simulink model "dry +no way scenario 1"  (R2025a)
settings: Solver=VariableStepAuto  StartTime=0.0  StopTime=10.0  RelTol=1e-3
libraries: SignalEditorBlockLib x5
settings Model: Creator=josik  LastModifiedBy=josik

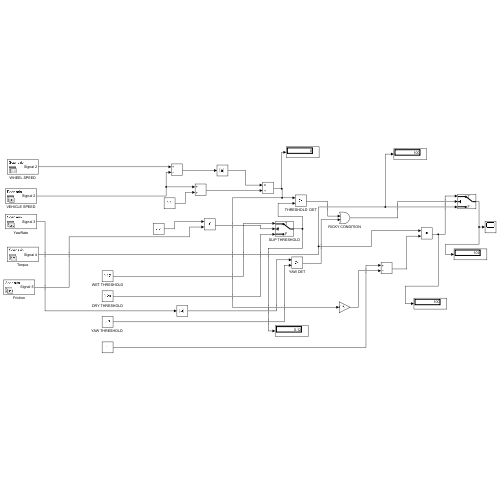
[thumbnail: Simulink's stored preview of the top-level diagram]
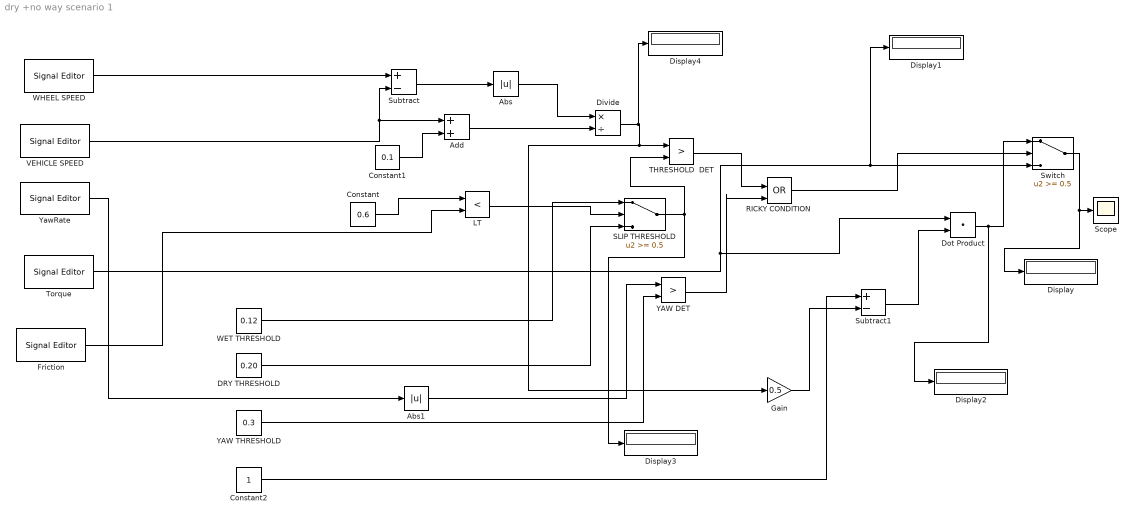
== system dry +no way scenario 1 ==
  Abs : Abs  SaturateOnIntegerOverflow=off
  Abs1 : Abs  SaturateOnIntegerOverflow=off
  Add : Sum
  Constant : Constant  Value=0.6
  Constant1 : Constant  Value=0.1
  Constant2 : Constant
  DRY THRESHOLD : Constant  Value=0.20
  Display{,1..4} (5 alike) : Display
  Divide : Product  Inputs=*/
  Dot Product : DotProduct  OutDataTypeStr=Inherit: Inherit via internal rule
  Friction : SignalEditorBlockLib/Signal Editor  FileName=signal 5 sc 3.mat  ActiveScenario=Scenario  ActiveSignal=Signal 5  IsBus=off  OutputBusObjectStr=Bus: BusObject  SampleTime=0  ZeroCross=off  OutputAfterFinalValue=Setting to zero  Unit=inherit  PreserveSignalName=on  ApplySigPropsToAllScenarios=on  ApplySigPropsToAllSignals=off  SignalPropertySource=Dialog parameters
  Gain : Gain  Gain=0.5
  LT : RelationalOperator  Operator=<  OutDataTypeStr=boolean  RndMeth=Simplest  InputSameDT=off
  RICKY CONDITION : Logic  Operator=OR  IconShape=distinctive  AllPortsSameDT=off  OutDataTypeStr=boolean
  SLIP THRESHOLD : Switch  Threshold=0.5  SaturateOnIntegerOverflow=off  InputSameDT=off
  Scope : Scope
      settings: ActiveDisplayYMinimum=0.26299668874172188  ActiveDisplayYMaximum=0.97077814569536425
  Subtract : Sum  Inputs=+-
  Subtract1 : Sum  Inputs=+-
  Switch : Switch  Threshold=0.5  SaturateOnIntegerOverflow=off  InputSameDT=off
  THRESHOLD  DET : RelationalOperator  Operator=>  OutDataTypeStr=boolean  RndMeth=Simplest  InputSameDT=off
  Torque : SignalEditorBlockLib/Signal Editor  FileName=signal 4 sc 3.mat  ActiveScenario=Scenario  ActiveSignal=Signal 4  IsBus=off  OutputBusObjectStr=Bus: BusObject  SampleTime=0  ZeroCross=off  OutputAfterFinalValue=Setting to zero  Unit=inherit  PreserveSignalName=on  ApplySigPropsToAllScenarios=on  ApplySigPropsToAllSignals=off  SignalPropertySource=Dialog parameters
  VEHICLE SPEED : SignalEditorBlockLib/Signal Editor  FileName=signal 2 sc 3.mat  ActiveScenario=Scenario  ActiveSignal=Signal 2  IsBus=off  OutputBusObjectStr=Bus: BusObject  SampleTime=0  ZeroCross=off  OutputAfterFinalValue=Setting to zero  Unit=inherit  PreserveSignalName=on  ApplySigPropsToAllScenarios=on  ApplySigPropsToAllSignals=off  SignalPropertySource=Dialog parameters
  WET THRESHOLD : Constant  Value=0.12
  WHEEL SPEED : SignalEditorBlockLib/Signal Editor  FileName=signal 2 sc 3.mat  ActiveScenario=Scenario  ActiveSignal=Signal 2  IsBus=off  OutputBusObjectStr=Bus: BusObject  SampleTime=0  ZeroCross=off  OutputAfterFinalValue=Setting to zero  Unit=inherit  PreserveSignalName=on  ApplySigPropsToAllScenarios=on  ApplySigPropsToAllSignals=off  SignalPropertySource=Dialog parameters
  YAW DET : RelationalOperator  Operator=>  OutDataTypeStr=boolean  RndMeth=Simplest  InputSameDT=off
  "YAW THRESHOLD " : Constant  Value=0.3
  YawRate : SignalEditorBlockLib/Signal Editor  FileName=signal 3 sc 3.mat  ActiveScenario=Scenario  ActiveSignal=Signal 3  IsBus=off  OutputBusObjectStr=Bus: BusObject  SampleTime=0  ZeroCross=off  OutputAfterFinalValue=Setting to zero  Unit=inherit  PreserveSignalName=on  ApplySigPropsToAllScenarios=on  ApplySigPropsToAllSignals=off  SignalPropertySource=Dialog parameters
  wires:
  Abs/1 -> Divide/1
  LT/1 -> SLIP THRESHOLD/2
  THRESHOLD  DET/1 -> RICKY CONDITION/1
  SLIP THRESHOLD/1 -> THRESHOLD  DET/2, Display3/1
  Constant/1 -> LT/1
  VEHICLE SPEED/1 -> Subtract/2, Add/1
  DRY THRESHOLD/1 -> SLIP THRESHOLD/3
  Gain/1 -> Subtract1/2
  Subtract1/1 -> Dot Product/2
  Constant1/1 -> Add/2
  YAW DET/1 -> RICKY CONDITION/2
  RICKY CONDITION/1 -> Switch/2
  WET THRESHOLD/1 -> SLIP THRESHOLD/1
  "YAW THRESHOLD "/1 -> YAW DET/2
  Add/1 -> Divide/2
  Subtract/1 -> Abs/1
  Switch/1 -> Display/1, Scope/1
  Divide/1 -> Display4/1, THRESHOLD  DET/1, Gain/1
  Torque/1 -> Switch/3, Display1/1, Dot Product/1
  YawRate/1 -> Abs1/1
  WHEEL SPEED/1 -> Subtract/1
  Dot Product/1 -> Display2/1, Switch/1
  Abs1/1 -> YAW DET/1
  Friction/1 -> LT/2
  Constant2/1 -> Subtract1/1
